simulink subsystem "Swerve_Drive_Module_sub"  (R2023b)
settings: Solver=VariableStepAuto  StartTime=0.0  StopTime=10.0  RelTol=1e-3
undefined symbols (not defined in the file): Drive_Motor_Control_Module_Angle_Error, Drive_Motor_Control_Scale_Factor, Wheel_Speed_to_Motor_Speed
libraries: Controls_Components_lib x6, simulink x2
settings Model: Creator=ander  LastModifiedBy=ander

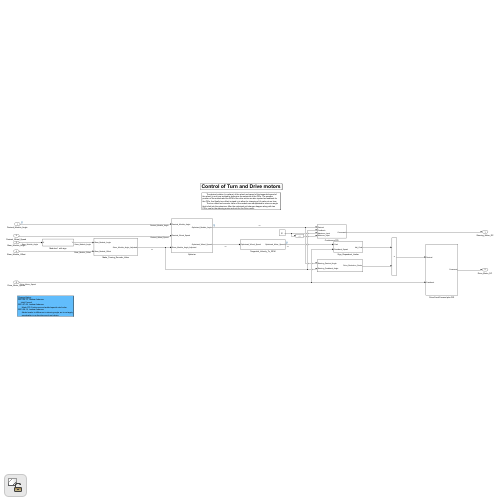
[thumbnail: Simulink's stored preview of the top-level diagram]
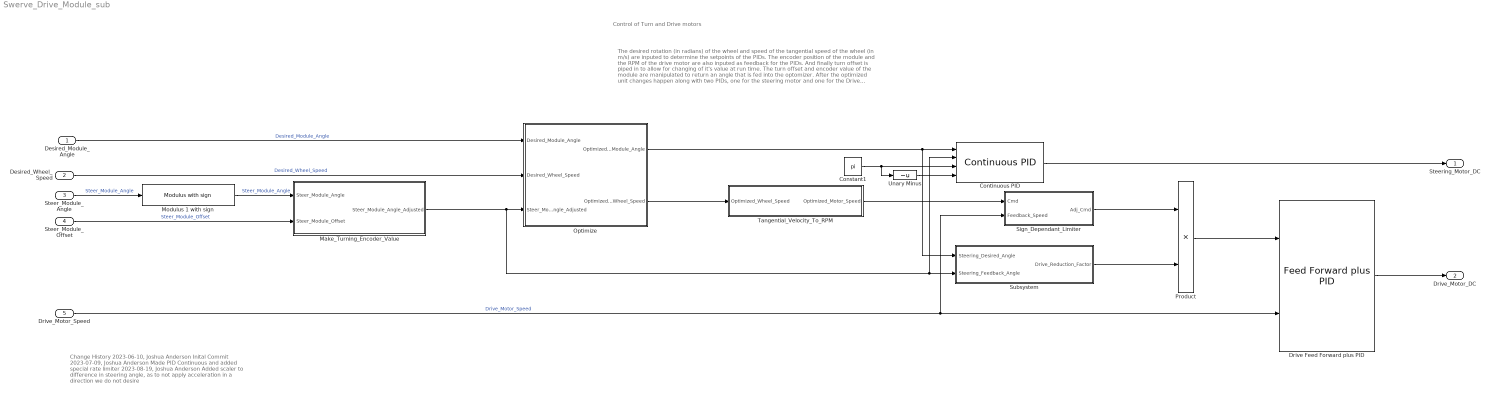
== system Swerve_Drive_Module_sub ==
  note: Control of Turn and Drive motors
  note: Change History
      | 2023-06-10, Joshua Anderson
      | Inital Commit
      | 2023-07-09, Joshua Anderson
      | Made PID Continuous and added special rate limiter
      | 2023-08-19, Joshua Anderson
      | Added scaler to difference in steering angle, as to not apply
      | acceleration in a direction we do not desire
  note: The desired rotation (in radians) of the wheel and speed of the tangential speed of the wheel (in m/s) are inputed to determine the setpoints of the PIDs. The encoder position of the module and the RPM of the drive motor are also inputed as feedback for the PIDs. And finally turn offset is piped in to allow for changing of it's value at run time.
      | 	The turn offset and encoder value of the module are manipulated to return an angle that is fed into the optomizer. After the optimized unit changes happen along with two PIDs, one for the steering motor and one for the Drive motor.
  Desired_Module_Angle : Inport  OutDataTypeStr=double  Unit=rad
  Desired_Wheel_Speed : Inport  Port=2  OutDataTypeStr=double  Unit=m/s
  Steer_Module_Angle : Inport  Port=3  OutDataTypeStr=double  Unit=rev
  Steer_Module_Offset : Inport  Port=4  OutDataTypeStr=double  Unit=rev
  Drive_Motor_Speed : Inport  Port=5  OutDataTypeStr=double  Unit=rpm
  Constant1 : Constant  Value=pi
  Continuous PID : Controls_Components_lib/Continuous PID  Gain_P=Steering_Motor_Control_P  Gain_I=Steering_Motor_Control_I  Gain_D=Steering_Motor_Control_D  FilterCoeff_D=Steering_Motor_Control_D_FilterCoeff  Limit_I_Upper=Steering_Motor_Control_I_UL  Limit_I_Lower=Steering_Motor_Control_I_LL  Limit_D_Upper=Steering_Motor_Control_D_UL  Limit_D_Lower=Steering_Motor_Control_D_LL  Limit_T_Upper=1  Limit_T_Lower=-1
  Drive Feed Forward plus PID : Controls_Components_lib/Feed Forward plus PID  Gain_FF=Drive_Motor_Control_FF  Gain_P=Drive_Motor_Control_P  Gain_I=Drive_Motor_Control_I  Gain_D=Drive_Motor_Control_D  FilterCoeff_D=Drive_Motor_Control_D_FilterCoeff  Limit_I_Upper=Drive_Motor_Control_I_UL  Limit_I_Lower=Drive_Motor_Control_I_LL  Limit_D_Upper=Drive_Motor_Control_D_UL  Limit_D_Lower=Drive_Motor_Control_D_LL  Limit_T_Upper=1  Limit_T_Lower=-1
  Make_Turning_Encoder_Value : Subsystem
  Modulus 1 with sign : Controls_Components_lib/Modulus with sign  Number=1
  Optimize : Subsystem
  Product : Product
  Sign_Dependant_Limiter : Subsystem  mask{Speed_Deadband=600}
      mask prompts: Speed_Deadband "Speed Deadband in RPM"
  Subsystem : Subsystem
  Tangential_Velocity_To_RPM : Subsystem
  Unary Minus : UnaryMinus
  Steering_Motor_DC : Outport  OutDataTypeStr=double  Unit=1
  Drive_Motor_DC : Outport  Port=2  OutDataTypeStr=double  Unit=1
  wires:
  Constant1/1 -> Unary Minus/1, Continuous PID/3
  Drive Feed Forward plus PID/1 -> Drive_Motor_DC/1
  Optimize/1(Optimized_Module_Angle) -> Continuous PID/1, Subsystem/1(Steering_Desired_Angle)
  Continuous PID/1 -> Steering_Motor_DC/1
  Steer_Module_Offset/1 -> Make_Turning_Encoder_Value/2(Steer_Module_Offset)  "Steer_Module_Offset"
  Make_Turning_Encoder_Value/1(Steer_Module_Angle_Adjusted) -> Subsystem/2(Steering_Feedback_Angle), Continuous PID/2, Optimize/3(Steer_Module_Angle_Adjusted)
  Steer_Module_Angle/1 -> Modulus 1 with sign/1  "Steer_Module_Angle"
  Tangential_Velocity_To_RPM/1(Optimized_Motor_Speed) -> Sign_Dependant_Limiter/1(Cmd)
  Optimize/2(Optimized_Wheel_Speed) -> Tangential_Velocity_To_RPM/1(Optimized_Wheel_Speed)
  Desired_Wheel_Speed/1 -> Optimize/2(Desired_Wheel_Speed)  "Desired_Wheel_Speed"
  Modulus 1 with sign/1 -> Make_Turning_Encoder_Value/1(Steer_Module_Angle)  "Steer_Module_Angle"
  Desired_Module_Angle/1 -> Optimize/1(Desired_Module_Angle)  "Desired_Module_Angle"
  Drive_Motor_Speed/1 -> Drive Feed Forward plus PID/2, Sign_Dependant_Limiter/2(Feedback_Speed)  "Drive_Motor_Speed"
  Sign_Dependant_Limiter/1(Adj_Cmd) -> Product/1
  Product/1 -> Drive Feed Forward plus PID/1
  Subsystem/1(Drive_Reduction_Factor) -> Product/2
  Unary Minus/1 -> Continuous PID/4

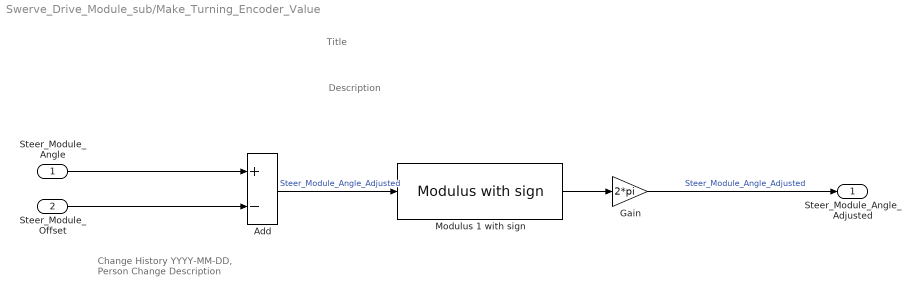
== system Swerve_Drive_Module_sub/Make_Turning_Encoder_Value ==
  note: Change History
      | YYYY-MM-DD, Person
      | Change Description
  note: Description
  note: Title
  Steer_Module_Angle : Inport  OutDataTypeStr=double  Unit=rev
  Steer_Module_Offset : Inport  Port=2  OutDataTypeStr=double  Unit=rev
  Add : Sum  Inputs=+-
  Gain : Gain  Gain=2*pi
  Modulus 1 with sign : Controls_Components_lib/Modulus with sign  Number=1
  Steer_Module_Angle_Adjusted : Outport  OutDataTypeStr=double  Unit=rad
  wires:
  Add/1 -> Modulus 1 with sign/1  "Steer_Module_Angle_Adjusted"
  Steer_Module_Offset/1 -> Add/2
  Steer_Module_Angle/1 -> Add/1
  Gain/1 -> Steer_Module_Angle_Adjusted/1  "Steer_Module_Angle_Adjusted"
  Modulus 1 with sign/1 -> Gain/1

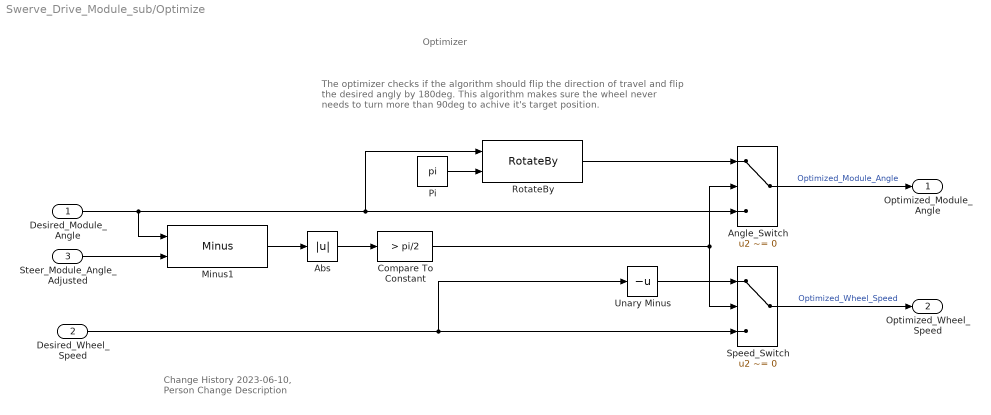
== system Swerve_Drive_Module_sub/Optimize ==
  note: The optimizer checks if the algorithm should flip the direction of travel and flip the desired angly by 180deg. This algorithm makes sure the wheel never needs to turn more than 90deg to achive it's target position.
  note: Change History
      | 2023-06-10, Person
      | Change Description
  note: Optimizer
  Desired_Module_Angle : Inport  OutDataTypeStr=double  Unit=rad
  Desired_Wheel_Speed : Inport  Port=2  OutDataTypeStr=double  Unit=m/s
  Steer_Module_Angle_Adjusted : Inport  Port=3  OutDataTypeStr=double  Unit=rad
  Abs : Abs  SaturateOnIntegerOverflow=off
  Angle_Switch : Switch  Criteria=u2 ~= 0  SaturateOnIntegerOverflow=off  InputSameDT=off
  Compare To Constant : simulink/Logic and Bit Operations/Compare To Constant  relop=>  const=pi/2  OutDataTypeStr=boolean
  Minus1 : Controls_Components_lib/Minus  SystemSampleTime=-1  VariantActivationTime=update diagram  AllowFlexibleInterface=on  Latency=0  AutoFrameSizeCalculation=off
  Pi : Constant  Value=pi  OutDataTypeStr=Inherit: Inherit via back propagation
  RotateBy : Controls_Components_lib/RotateBy  SystemSampleTime=-1  VariantActivationTime=update diagram  AllowFlexibleInterface=on  Latency=0  AutoFrameSizeCalculation=off
  Speed_Switch : Switch  Criteria=u2 ~= 0  SaturateOnIntegerOverflow=off  InputSameDT=off
  Unary Minus : UnaryMinus
  Optimized_Module_Angle : Outport  OutDataTypeStr=double  Unit=rad
  Optimized_Wheel_Speed : Outport  Port=2  OutDataTypeStr=double  Unit=m/s
  wires:
  Desired_Module_Angle/1 -> Minus1/1, RotateBy/1, Angle_Switch/3
  Steer_Module_Angle_Adjusted/1 -> Minus1/2
  Minus1/1 -> Abs/1
  Abs/1 -> Compare To Constant/1
  Desired_Wheel_Speed/1 -> Unary Minus/1, Speed_Switch/3
  Compare To Constant/1 -> Angle_Switch/2, Speed_Switch/2
  Unary Minus/1 -> Speed_Switch/1
  Pi/1 -> RotateBy/2
  Angle_Switch/1 -> Optimized_Module_Angle/1  "Optimized_Module_Angle"
  Speed_Switch/1 -> Optimized_Wheel_Speed/1  "Optimized_Wheel_Speed"
  RotateBy/1 -> Angle_Switch/1

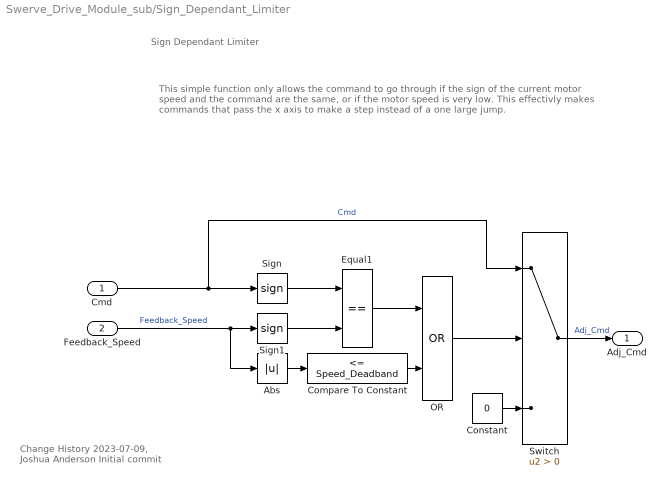
== system Swerve_Drive_Module_sub/Sign_Dependant_Limiter ==
  note: Sign Dependant Limiter
  note: Change History
      | 2023-07-09, Joshua Anderson
      | Initial commit
  note: This simple function only allows the command to go through if the sign of the current motor speed and the command are the same, or if the motor speed is very low. This effectivly makes commands that pass the x axis to make a step instead of a one large jump.
  Cmd : Inport
  Feedback_Speed : Inport  Port=2
  Abs : Abs  SaturateOnIntegerOverflow=off
  Compare To Constant : simulink/Logic and Bit Operations/Compare To Constant  relop=<=  const=Speed_Deadband  OutDataTypeStr=boolean
  Constant : Constant  Value=0
  Equal1 : RelationalOperator  Operator===  OutDataTypeStr=boolean  RndMeth=Simplest  InputSameDT=off
  OR : Logic  Operator=OR  AllPortsSameDT=off  OutDataTypeStr=boolean
  Sign : Signum
  Sign1 : Signum
  Switch : Switch  Criteria=u2 > Threshold  SaturateOnIntegerOverflow=off  InputSameDT=off
  Adj_Cmd : Outport
  wires:
  Compare To Constant/1 -> OR/2
  Sign/1 -> Equal1/1
  Constant/1 -> Switch/3
  Equal1/1 -> OR/1
  Cmd/1 -> Sign/1, Switch/1  "Cmd"
  Sign1/1 -> Equal1/2
  Switch/1 -> Adj_Cmd/1  "Adj_Cmd"
  Feedback_Speed/1 -> Sign1/1, Abs/1  "Feedback_Speed"
  Abs/1 -> Compare To Constant/1
  OR/1 -> Switch/2

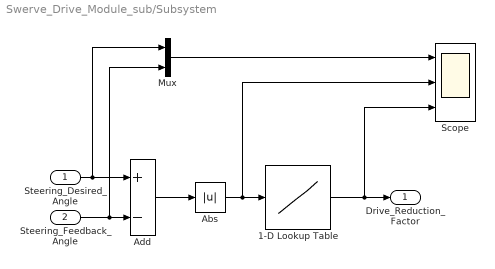
== system Swerve_Drive_Module_sub/Subsystem ==
  Steering_Desired_Angle : Inport
  Steering_Feedback_Angle : Inport  Port=2
  1-D Lookup Table : Lookup_n-D  NumberOfTableDimensions=1  BreakpointsForDimension1=Drive_Motor_Control_Module_Angle_Error  Table=Drive_Motor_Control_Scale_Factor  ExtrapMethod=Clip  InternalRulePriority=Speed  RndMeth=Simplest
  Abs : Abs  SaturateOnIntegerOverflow=off
  Add : Sum  Inputs=+-
  Mux : Mux  Inputs=2
  Scope : Scope  NumInputPorts=3
  Drive_Reduction_Factor : Outport
  wires:
  Mux/1 -> Scope/1
  1-D Lookup Table/1 -> Drive_Reduction_Factor/1, Scope/3
  Abs/1 -> 1-D Lookup Table/1, Scope/2
  Add/1 -> Abs/1
  Steering_Feedback_Angle/1 -> Add/2, Mux/2
  Steering_Desired_Angle/1 -> Add/1, Mux/1

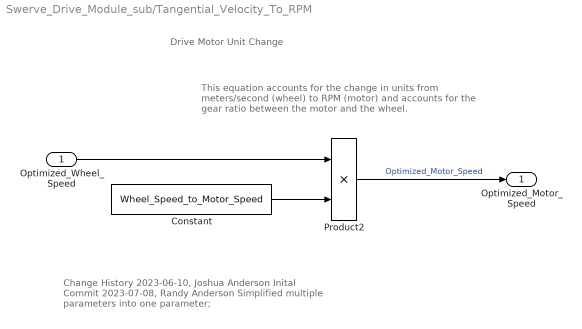
== system Swerve_Drive_Module_sub/Tangential_Velocity_To_RPM ==
  note: This equation accounts for the change in units from meters/second (wheel) to RPM (motor) and accounts for the gear ratio between the motor and the wheel.
  note: Change History
      | 2023-06-10, Joshua Anderson
      | Inital Commit
      | 2023-07-08, Randy Anderson
      | Simplified multiple parameters into one parameter;
  note: Drive Motor Unit Change
  Optimized_Wheel_Speed : Inport  Unit=m/s
  Constant : Constant  Value=Wheel_Speed_to_Motor_Speed
  Product2 : Product
  Optimized_Motor_Speed : Outport  Unit=rpm
  wires:
  Product2/1 -> Optimized_Motor_Speed/1  "Optimized_Motor_Speed"
  Optimized_Wheel_Speed/1 -> Product2/1
  Constant/1 -> Product2/2
